simulink model "snap2_f_200msps_64i_4096c"  (R2019a)
settings: Solver=VariableStepDiscrete  StartTime=0.0  StopTime=10.0  RelTol=1e-3
undefined symbols (not defined in the file or in its folder): datetime, posixtime
libraries: xbsIndex_r4 x21354, casper_library_misc x297, casper_library_delays x19, xps_library x14, casper_library_sources x4
(part 8 of 217)

== system snap2_f_200msps_64i_4096c/version ==
  Concat : xbsIndex_r4/Concat  num_inputs=4  dbl_ovrd=off  block_type=concat
  Constant : xbsIndex_r4/Constant  const=ver_maj  gui_display_data_type=Fixed-point  arith_type=Unsigned  n_bits=8  bin_pt=0  preci_type=Single  exp_width=8  frac_width=24  explicit_period=on  period=1  equ=P=C  opselect=C  inp2=PCIN>>17  opr=+  inp1=P  carry=CIN  dbl_ovrd=off  block_type=constant
  Constant1 : xbsIndex_r4/Constant  const=ver_min  gui_display_data_type=Fixed-point  arith_type=Unsigned  n_bits=8  bin_pt=0  preci_type=Single  exp_width=8  frac_width=24  explicit_period=on  period=1  equ=P=C  opselect=C  inp2=PCIN>>17  opr=+  inp1=P  carry=CIN  dbl_ovrd=off  block_type=constant
  Constant2 : xbsIndex_r4/Constant  const=ver_rev  gui_display_data_type=Fixed-point  arith_type=Unsigned  n_bits=8  bin_pt=0  preci_type=Single  exp_width=8  frac_width=24  explicit_period=on  period=1  equ=P=C  opselect=C  inp2=PCIN>>17  opr=+  inp1=P  carry=CIN  dbl_ovrd=off  block_type=constant
  Constant3 : xbsIndex_r4/Constant  const=ver_bugfix  gui_display_data_type=Fixed-point  arith_type=Unsigned  n_bits=8  bin_pt=0  preci_type=Single  exp_width=8  frac_width=24  explicit_period=on  period=1  equ=P=C  opselect=C  inp2=PCIN>>17  opr=+  inp1=P  carry=CIN  dbl_ovrd=off  block_type=constant
  Terminator1 : Terminator
  Terminator2 : Terminator
  timestamp : Subsystem  Tag=xps:sw_reg  AncestorBlock=xps_library/Memory/software_register  mask(swreg){io_dir=To Processor, io_delay=0, init_val=0, sample_period=1, names=reg, bitwidths=32, bin_pts=0, arith_types=0, sim_port=on, show_format=off, desc_str=Unix timestamp, in integer seconds, when firmware was last compiled.}
      mask prompts: io_dir "I/O direction"; io_delay "I/O delay"; init_val "Initial Value"; sample_period "Sample period"; names "Bitfield names [msb...lsb]"; bitwidths "Bitfield widths"; bin_pts "Bitfield binary pts"; arith_types "Bitfield types, ufix=0, fix=1, bool=2"; sim_port "Provide sim input/output?"; show_format "Print format string?"; desc_str "Description"
      mask help: A 32-bit software-accessible register. Can be divided into bitfields of varying widths and types using the fields in the block mask.
      mask init:
      | swreg_init(gcb)
      settings: AttributesFormatString=1output
      mask TypeOptions io_dir: To Processor | From Processor
      mask Callback io_dir:
      | mask_enables = get_param(gcb, 'MaskEnables');
      | mask_names = get_param(gcb, 'MaskNames');
      | if strcmp(get_param(gcb, 'io_dir'), 'To Processor'),
      |     mask_enables{ismember(mask_names, 'sample_period')} = 'off';
      | else
      |     mask_enables{ismember(mask_names, 'sample_period')} = 'on';
      | end
      | set_param(gcb, 'MaskEnables', mask_enables);
      mask DialogControl ParameterTabVar0 Prompt: Setup
  unix_time : xbsIndex_r4/Constant  const=round(posixtime(datetime('now')))  gui_display_data_type=Fixed-point  arith_type=Unsigned  n_bits=32  bin_pt=0  preci_type=Single  exp_width=8  frac_width=24  explicit_period=on  period=1  equ=P=C  opselect=C  inp2=PCIN>>17  opr=+  inp1=P  carry=CIN  dbl_ovrd=off  block_type=constant
  version : Subsystem  Tag=xps:sw_reg  AncestorBlock=xps_library/Memory/software_register  mask(swreg){io_dir=To Processor, io_delay=0, init_val=0, sample_period=1, names=reg, bitwidths=32, bin_pts=0, arith_types=0, sim_port=on, show_format=off, desc_str=|}
      mask desc_str=|
      | Version register. Bits ``[31:24]``: major version. Bits
      | ``[23:16]``: minor version. Bits ``[15:8]``: revision.
      | Bits ``[7:0]``: buxfix.
      mask prompts: io_dir "I/O direction"; io_delay "I/O delay"; init_val "Initial Value"; sample_period "Sample period"; names "Bitfield names [msb...lsb]"; bitwidths "Bitfield widths"; bin_pts "Bitfield binary pts"; arith_types "Bitfield types, ufix=0, fix=1, bool=2"; sim_port "Provide sim input/output?"; show_format "Print format string?"; desc_str "Description"
      mask help: A 32-bit software-accessible register. Can be divided into bitfields of varying widths and types using the fields in the block mask.
      mask init:
      | swreg_init(gcb)
      settings: AttributesFormatString=1output
      mask TypeOptions io_dir: To Processor | From Processor
      mask Callback io_dir:
      | mask_enables = get_param(gcb, 'MaskEnables');
      | mask_names = get_param(gcb, 'MaskNames');
      | if strcmp(get_param(gcb, 'io_dir'), 'To Processor'),
      |     mask_enables{ismember(mask_names, 'sample_period')} = 'off';
      | else
      |     mask_enables{ismember(mask_names, 'sample_period')} = 'on';
      | end
      | set_param(gcb, 'MaskEnables', mask_enables);
      mask DialogControl ParameterTabVar0 Prompt: Setup
  wires:
  Constant1/1 -> Concat/2
  Concat/1 -> version/1(out_reg)
  Constant/1 -> Concat/1
  version/1(sim_out_reg) -> Terminator1/1
  Constant2/1 -> Concat/3
  Constant3/1 -> Concat/4
  timestamp/1(sim_out_reg) -> Terminator2/1
  unix_time/1 -> timestamp/1(out_reg)

== system snap2_f_200msps_64i_4096c/adc/bus_create ==
  in1 : Inport
  in2 : Inport  Port=2
  in3 : Inport  Port=3
  in4 : Inport  Port=4
  in5 : Inport  Port=5
  in6 : Inport  Port=6
  in7 : Inport  Port=7
  in8 : Inport  Port=8
  in9 : Inport  Port=9
  in10 : Inport  Port=10
  in11 : Inport  Port=11
  in12 : Inport  Port=12
  in13 : Inport  Port=13
  in14 : Inport  Port=14
  in15 : Inport  Port=15
  in16 : Inport  Port=16
  in17 : Inport  Port=17
  in18 : Inport  Port=18
  in19 : Inport  Port=19
  in20 : Inport  Port=20
  in21 : Inport  Port=21
  in22 : Inport  Port=22
  in23 : Inport  Port=23
  in24 : Inport  Port=24
  in25 : Inport  Port=25
  in26 : Inport  Port=26
  in27 : Inport  Port=27
  in28 : Inport  Port=28
  in29 : Inport  Port=29
  in30 : Inport  Port=30
  in31 : Inport  Port=31
  in32 : Inport  Port=32
  in33 : Inport  Port=33
  in34 : Inport  Port=34
  in35 : Inport  Port=35
  in36 : Inport  Port=36
  in37 : Inport  Port=37
  in38 : Inport  Port=38
  in39 : Inport  Port=39
  in40 : Inport  Port=40
  in41 : Inport  Port=41
  in42 : Inport  Port=42
  in43 : Inport  Port=43
  in44 : Inport  Port=44
  in45 : Inport  Port=45
  in46 : Inport  Port=46
  in47 : Inport  Port=47
  in48 : Inport  Port=48
  in49 : Inport  Port=49
  in50 : Inport  Port=50
  in51 : Inport  Port=51
  in52 : Inport  Port=52
  in53 : Inport  Port=53
  in54 : Inport  Port=54
  in55 : Inport  Port=55
  in56 : Inport  Port=56
  in57 : Inport  Port=57
  in58 : Inport  Port=58
  in59 : Inport  Port=59
  in60 : Inport  Port=60
  in61 : Inport  Port=61
  in62 : Inport  Port=62
  in63 : Inport  Port=63
  in64 : Inport  Port=64
  concatenate : xbsIndex_r4/Concat  num_inputs=64  dbl_ovrd=off  block_type=concat
  reinterpret{1..64} (64 alike) : xbsIndex_r4/Reinterpret  force_arith_type=on  arith_type=Unsigned  force_bin_pt=on  bin_pt=0  block_type=reinterpret
      reinterpret1 settings: infoedit="Changes signal type without altering the binary representation.   You can changed the signal between signed and unsigned, and relocate the binary point.<br><br>Hardware notes: In hardware this block costs nothing.<br><br>Example:  Suppose the input is 6 bits wide, signed, with 2 fractional bits, and the output is forced to unsigned with 0 fractional bits.  Then an input of -2.0 (1110.00 in binary 2's complement) becomes an output of 56 (111000 in binary)."
      reinterpret2 settings: infoedit="Changes signal type without altering the binary representation.   You can changed the signal between signed and unsigned, and relocate the binary point.<br><br>Hardware notes: In hardware this block costs nothing.<br><br>Example:  Suppose the input is 6 bits wide, signed, with 2 fractional bits, and the output is forced to unsigned with 0 fractional bits.  Then an input of -2.0 (1110.00 in binary 2's complement) becomes an output of 56 (111000 in binary)."
  bus_out : Outport
  wires:
  concatenate/1 -> bus_out/1
  in1/1 -> reinterpret1/1
  reinterpret1/1 -> concatenate/1
  in2/1 -> reinterpret2/1
  reinterpret2/1 -> concatenate/2
  in3/1 -> reinterpret3/1
  reinterpret3/1 -> concatenate/3
  in4/1 -> reinterpret4/1
  reinterpret4/1 -> concatenate/4
  in5/1 -> reinterpret5/1
  reinterpret5/1 -> concatenate/5
  in6/1 -> reinterpret6/1
  reinterpret6/1 -> concatenate/6
  in7/1 -> reinterpret7/1
  reinterpret7/1 -> concatenate/7
  in8/1 -> reinterpret8/1
  reinterpret8/1 -> concatenate/8
  in9/1 -> reinterpret9/1
  reinterpret9/1 -> concatenate/9
  in10/1 -> reinterpret10/1
  reinterpret10/1 -> concatenate/10
  in11/1 -> reinterpret11/1
  reinterpret11/1 -> concatenate/11
  in12/1 -> reinterpret12/1
  reinterpret12/1 -> concatenate/12
  in13/1 -> reinterpret13/1
  reinterpret13/1 -> concatenate/13
  in14/1 -> reinterpret14/1
  reinterpret14/1 -> concatenate/14
  in15/1 -> reinterpret15/1
  reinterpret15/1 -> concatenate/15
  in16/1 -> reinterpret16/1
  reinterpret16/1 -> concatenate/16
  in17/1 -> reinterpret17/1
  reinterpret17/1 -> concatenate/17
  in18/1 -> reinterpret18/1
  reinterpret18/1 -> concatenate/18
  in19/1 -> reinterpret19/1
  reinterpret19/1 -> concatenate/19
  in20/1 -> reinterpret20/1
  reinterpret20/1 -> concatenate/20
  in21/1 -> reinterpret21/1
  reinterpret21/1 -> concatenate/21
  in22/1 -> reinterpret22/1
  reinterpret22/1 -> concatenate/22
  in23/1 -> reinterpret23/1
  reinterpret23/1 -> concatenate/23
  in24/1 -> reinterpret24/1
  reinterpret24/1 -> concatenate/24
  in25/1 -> reinterpret25/1
  reinterpret25/1 -> concatenate/25
  in26/1 -> reinterpret26/1
  reinterpret26/1 -> concatenate/26
  in27/1 -> reinterpret27/1
  reinterpret27/1 -> concatenate/27
  in28/1 -> reinterpret28/1
  reinterpret28/1 -> concatenate/28
  in29/1 -> reinterpret29/1
  reinterpret29/1 -> concatenate/29
  in30/1 -> reinterpret30/1
  reinterpret30/1 -> concatenate/30
  in31/1 -> reinterpret31/1
  reinterpret31/1 -> concatenate/31
  in32/1 -> reinterpret32/1
  reinterpret32/1 -> concatenate/32
  in33/1 -> reinterpret33/1
  reinterpret33/1 -> concatenate/33
  in34/1 -> reinterpret34/1
  reinterpret34/1 -> concatenate/34
  in35/1 -> reinterpret35/1
  reinterpret35/1 -> concatenate/35
  in36/1 -> reinterpret36/1
  reinterpret36/1 -> concatenate/36
  in37/1 -> reinterpret37/1
  reinterpret37/1 -> concatenate/37
  in38/1 -> reinterpret38/1
  reinterpret38/1 -> concatenate/38
  in39/1 -> reinterpret39/1
  reinterpret39/1 -> concatenate/39
  in40/1 -> reinterpret40/1
  reinterpret40/1 -> concatenate/40
  in41/1 -> reinterpret41/1
  reinterpret41/1 -> concatenate/41
  in42/1 -> reinterpret42/1
  reinterpret42/1 -> concatenate/42
  in43/1 -> reinterpret43/1
  reinterpret43/1 -> concatenate/43
  in44/1 -> reinterpret44/1
  reinterpret44/1 -> concatenate/44
  in45/1 -> reinterpret45/1
  reinterpret45/1 -> concatenate/45
  in46/1 -> reinterpret46/1
  reinterpret46/1 -> concatenate/46
  in47/1 -> reinterpret47/1
  reinterpret47/1 -> concatenate/47
  in48/1 -> reinterpret48/1
  reinterpret48/1 -> concatenate/48
  in49/1 -> reinterpret49/1
  reinterpret49/1 -> concatenate/49
  in50/1 -> reinterpret50/1
  reinterpret50/1 -> concatenate/50
  in51/1 -> reinterpret51/1
  reinterpret51/1 -> concatenate/51
  in52/1 -> reinterpret52/1
  reinterpret52/1 -> concatenate/52
  in53/1 -> reinterpret53/1
  reinterpret53/1 -> concatenate/53
  in54/1 -> reinterpret54/1
  reinterpret54/1 -> concatenate/54
  in55/1 -> reinterpret55/1
  reinterpret55/1 -> concatenate/55
  in56/1 -> reinterpret56/1
  reinterpret56/1 -> concatenate/56
  in57/1 -> reinterpret57/1
  reinterpret57/1 -> concatenate/57
  in58/1 -> reinterpret58/1
  reinterpret58/1 -> concatenate/58
  in59/1 -> reinterpret59/1
  reinterpret59/1 -> concatenate/59
  in60/1 -> reinterpret60/1
  reinterpret60/1 -> concatenate/60
  in61/1 -> reinterpret61/1
  reinterpret61/1 -> concatenate/61
  in62/1 -> reinterpret62/1
  reinterpret62/1 -> concatenate/62
  in63/1 -> reinterpret63/1
  reinterpret63/1 -> concatenate/63
  in64/1 -> reinterpret64/1
  reinterpret64/1 -> concatenate/64

== system snap2_f_200msps_64i_4096c/adc/fmc0 ==
  a1_sim : Inport
  a2_sim : Inport  Port=2
  a3_sim : Inport  Port=3
  a4_sim : Inport  Port=4
  b1_sim : Inport  Port=5
  b2_sim : Inport  Port=6
  b3_sim : Inport  Port=7
  b4_sim : Inport  Port=8
  c1_sim : Inport  Port=9
  c2_sim : Inport  Port=10
  c3_sim : Inport  Port=11
  c4_sim : Inport  Port=12
  d1_sim : Inport  Port=13
  d2_sim : Inport  Port=14
  d3_sim : Inport  Port=15
  d4_sim : Inport  Port=16
  e1_sim : Inport  Port=17
  e2_sim : Inport  Port=18
  e3_sim : Inport  Port=19
  e4_sim : Inport  Port=20
  f1_sim : Inport  Port=21
  f2_sim : Inport  Port=22
  f3_sim : Inport  Port=23
  f4_sim : Inport  Port=24
  g1_sim : Inport  Port=25
  g2_sim : Inport  Port=26
  g3_sim : Inport  Port=27
  g4_sim : Inport  Port=28
  h1_sim : Inport  Port=29
  h2_sim : Inport  Port=30
  h3_sim : Inport  Port=31
  h4_sim : Inport  Port=32
  sync : Inport  Port=33
  snapshot_trig : Inport  Port=34
  sim_sync_out : Inport  Port=35
  rst : Inport  Port=36
  rst_term : Terminator
  snap2_f_200msps_64i_4096c_adc_fmc0_a{1..4} (4 alike) : xbsIndex_r4/Gateway In  gui_display_data_type=Fixed-point  arith_type="Signed  (2's comp)"  n_bits=10  bin_pt=9  preci_type=Single  exp_width=8  frac_width=24  rows=1  columns=1  quantization="Round  (unbiased: +/- Inf)"  overflow=Saturate  period=1  UseAsADC=off  ADCChannel='1'  interface=None  automatic_assignment=on  address_offset=hex2dec('00')  intf_name=''  intf_description=''  default_value=0  timing_constraint=None  locs_specified=off  LOCs={}  io_standard={}  inherit_from_input=off  hdl_port=on  dbl_ovrd=off  block_type=gatewayin
  snap2_f_200msps_64i_4096c_adc_fmc0_adc_rst : xbsIndex_r4/Gateway Out  inherit_from_input=off  hdl_port=on  rows=1  columns=1  UseAsDAC=off  DACChannel='1'  interface=None  automatic_assignment=on  address_offset=hex2dec('00')  intf_name=''  intf_description=''  timing_constraint=None  locs_specified=off  LOCs={}  io_standard={}  block_type=gatewayout
  snap2_f_200msps_64i_4096c_adc_fmc0_adc_sync : xbsIndex_r4/Gateway Out  inherit_from_input=off  hdl_port=on  rows=1  columns=1  UseAsDAC=off  DACChannel='1'  interface=None  automatic_assignment=on  address_offset=hex2dec('00')  intf_name=''  intf_description=''  timing_constraint=None  locs_specified=off  LOCs={}  io_standard={}  block_type=gatewayout
  snap2_f_200msps_64i_4096c_adc_fmc0_adc_sync_out : xbsIndex_r4/Gateway In  gui_display_data_type=Fixed-point  arith_type=Boolean  n_bits=16  bin_pt=14  preci_type=Single  exp_width=8  frac_width=24  rows=1  columns=1  quantization="Round  (unbiased: +/- Inf)"  overflow=Saturate  period=1  UseAsADC=off  ADCChannel='1'  interface=None  automatic_assignment=on  address_offset=hex2dec('00')  intf_name=''  intf_description=''  default_value=0  timing_constraint=None  locs_specified=off  LOCs={}  io_standard={}  inherit_from_input=off  hdl_port=on  dbl_ovrd=off  block_type=gatewayin
  snap2_f_200msps_64i_4096c_adc_fmc0_b{1..4} (4 alike) : xbsIndex_r4/Gateway In  gui_display_data_type=Fixed-point  arith_type="Signed  (2's comp)"  n_bits=10  bin_pt=9  preci_type=Single  exp_width=8  frac_width=24  rows=1  columns=1  quantization="Round  (unbiased: +/- Inf)"  overflow=Saturate  period=1  UseAsADC=off  ADCChannel='1'  interface=None  automatic_assignment=on  address_offset=hex2dec('00')  intf_name=''  intf_description=''  default_value=0  timing_constraint=None  locs_specified=off  LOCs={}  io_standard={}  inherit_from_input=off  hdl_port=on  dbl_ovrd=off  block_type=gatewayin
  snap2_f_200msps_64i_4096c_adc_fmc0_c{1..4} (4 alike) : xbsIndex_r4/Gateway In  gui_display_data_type=Fixed-point  arith_type="Signed  (2's comp)"  n_bits=10  bin_pt=9  preci_type=Single  exp_width=8  frac_width=24  rows=1  columns=1  quantization="Round  (unbiased: +/- Inf)"  overflow=Saturate  period=1  UseAsADC=off  ADCChannel='1'  interface=None  automatic_assignment=on  address_offset=hex2dec('00')  intf_name=''  intf_description=''  default_value=0  timing_constraint=None  locs_specified=off  LOCs={}  io_standard={}  inherit_from_input=off  hdl_port=on  dbl_ovrd=off  block_type=gatewayin
  snap2_f_200msps_64i_4096c_adc_fmc0_d{1..4} (4 alike) : xbsIndex_r4/Gateway In  gui_display_data_type=Fixed-point  arith_type="Signed  (2's comp)"  n_bits=10  bin_pt=9  preci_type=Single  exp_width=8  frac_width=24  rows=1  columns=1  quantization="Round  (unbiased: +/- Inf)"  overflow=Saturate  period=1  UseAsADC=off  ADCChannel='1'  interface=None  automatic_assignment=on  address_offset=hex2dec('00')  intf_name=''  intf_description=''  default_value=0  timing_constraint=None  locs_specified=off  LOCs={}  io_standard={}  inherit_from_input=off  hdl_port=on  dbl_ovrd=off  block_type=gatewayin
  snap2_f_200msps_64i_4096c_adc_fmc0_e{1..4} (4 alike) : xbsIndex_r4/Gateway In  gui_display_data_type=Fixed-point  arith_type="Signed  (2's comp)"  n_bits=10  bin_pt=9  preci_type=Single  exp_width=8  frac_width=24  rows=1  columns=1  quantization="Round  (unbiased: +/- Inf)"  overflow=Saturate  period=1  UseAsADC=off  ADCChannel='1'  interface=None  automatic_assignment=on  address_offset=hex2dec('00')  intf_name=''  intf_description=''  default_value=0  timing_constraint=None  locs_specified=off  LOCs={}  io_standard={}  inherit_from_input=off  hdl_port=on  dbl_ovrd=off  block_type=gatewayin
  snap2_f_200msps_64i_4096c_adc_fmc0_f{1..4} (4 alike) : xbsIndex_r4/Gateway In  gui_display_data_type=Fixed-point  arith_type="Signed  (2's comp)"  n_bits=10  bin_pt=9  preci_type=Single  exp_width=8  frac_width=24  rows=1  columns=1  quantization="Round  (unbiased: +/- Inf)"  overflow=Saturate  period=1  UseAsADC=off  ADCChannel='1'  interface=None  automatic_assignment=on  address_offset=hex2dec('00')  intf_name=''  intf_description=''  default_value=0  timing_constraint=None  locs_specified=off  LOCs={}  io_standard={}  inherit_from_input=off  hdl_port=on  dbl_ovrd=off  block_type=gatewayin
  snap2_f_200msps_64i_4096c_adc_fmc0_g{1..4} (4 alike) : xbsIndex_r4/Gateway In  gui_display_data_type=Fixed-point  arith_type="Signed  (2's comp)"  n_bits=10  bin_pt=9  preci_type=Single  exp_width=8  frac_width=24  rows=1  columns=1  quantization="Round  (unbiased: +/- Inf)"  overflow=Saturate  period=1  UseAsADC=off  ADCChannel='1'  interface=None  automatic_assignment=on  address_offset=hex2dec('00')  intf_name=''  intf_description=''  default_value=0  timing_constraint=None  locs_specified=off  LOCs={}  io_standard={}  inherit_from_input=off  hdl_port=on  dbl_ovrd=off  block_type=gatewayin
  snap2_f_200msps_64i_4096c_adc_fmc0_h{1..4} (4 alike) : xbsIndex_r4/Gateway In  gui_display_data_type=Fixed-point  arith_type="Signed  (2's comp)"  n_bits=10  bin_pt=9  preci_type=Single  exp_width=8  frac_width=24  rows=1  columns=1  quantization="Round  (unbiased: +/- Inf)"  overflow=Saturate  period=1  UseAsADC=off  ADCChannel='1'  interface=None  automatic_assignment=on  address_offset=hex2dec('00')  intf_name=''  intf_description=''  default_value=0  timing_constraint=None  locs_specified=off  LOCs={}  io_standard={}  inherit_from_input=off  hdl_port=on  dbl_ovrd=off  block_type=gatewayin
  snap2_f_200msps_64i_4096c_adc_fmc0_snapshot_ext_trigger : xbsIndex_r4/Gateway Out  inherit_from_input=off  hdl_port=on  rows=1  columns=1  UseAsDAC=off  DACChannel='1'  interface=None  automatic_assignment=on  address_offset=hex2dec('00')  intf_name=''  intf_description=''  timing_constraint=None  locs_specified=off  LOCs={}  io_standard={}  block_type=gatewayout
  snapshot_trig_term : Terminator
  sync_term : Terminator
  a1 : Outport
  a2 : Outport  Port=2
  a3 : Outport  Port=3
  a4 : Outport  Port=4
  b1 : Outport  Port=5
  b2 : Outport  Port=6
  b3 : Outport  Port=7
  b4 : Outport  Port=8
  c1 : Outport  Port=9
  c2 : Outport  Port=10
  c3 : Outport  Port=11
  c4 : Outport  Port=12
  d1 : Outport  Port=13
  d2 : Outport  Port=14
  d3 : Outport  Port=15
  d4 : Outport  Port=16
  e1 : Outport  Port=17
  e2 : Outport  Port=18
  e3 : Outport  Port=19
  e4 : Outport  Port=20
  f1 : Outport  Port=21
  f2 : Outport  Port=22
  f3 : Outport  Port=23
  f4 : Outport  Port=24
  g1 : Outport  Port=25
  g2 : Outport  Port=26
  g3 : Outport  Port=27
  g4 : Outport  Port=28
  h1 : Outport  Port=29
  h2 : Outport  Port=30
  h3 : Outport  Port=31
  h4 : Outport  Port=32
  sync_out : Outport  Port=33
  wires:
  a1_sim/1 -> snap2_f_200msps_64i_4096c_adc_fmc0_a1/1
  snap2_f_200msps_64i_4096c_adc_fmc0_a1/1 -> a1/1  "a1"
  a2_sim/1 -> snap2_f_200msps_64i_4096c_adc_fmc0_a2/1
  snap2_f_200msps_64i_4096c_adc_fmc0_a2/1 -> a2/1  "a2"
  a3_sim/1 -> snap2_f_200msps_64i_4096c_adc_fmc0_a3/1
  snap2_f_200msps_64i_4096c_adc_fmc0_a3/1 -> a3/1  "a3"
  a4_sim/1 -> snap2_f_200msps_64i_4096c_adc_fmc0_a4/1
  snap2_f_200msps_64i_4096c_adc_fmc0_a4/1 -> a4/1  "a4"
  b1_sim/1 -> snap2_f_200msps_64i_4096c_adc_fmc0_b1/1
  snap2_f_200msps_64i_4096c_adc_fmc0_b1/1 -> b1/1  "b1"
  b2_sim/1 -> snap2_f_200msps_64i_4096c_adc_fmc0_b2/1
  snap2_f_200msps_64i_4096c_adc_fmc0_b2/1 -> b2/1  "b2"
  b3_sim/1 -> snap2_f_200msps_64i_4096c_adc_fmc0_b3/1
  snap2_f_200msps_64i_4096c_adc_fmc0_b3/1 -> b3/1  "b3"
  b4_sim/1 -> snap2_f_200msps_64i_4096c_adc_fmc0_b4/1
  snap2_f_200msps_64i_4096c_adc_fmc0_b4/1 -> b4/1  "b4"
  c1_sim/1 -> snap2_f_200msps_64i_4096c_adc_fmc0_c1/1
  snap2_f_200msps_64i_4096c_adc_fmc0_c1/1 -> c1/1  "c1"
  c2_sim/1 -> snap2_f_200msps_64i_4096c_adc_fmc0_c2/1
  snap2_f_200msps_64i_4096c_adc_fmc0_c2/1 -> c2/1  "c2"
  c3_sim/1 -> snap2_f_200msps_64i_4096c_adc_fmc0_c3/1
  snap2_f_200msps_64i_4096c_adc_fmc0_c3/1 -> c3/1  "c3"
  c4_sim/1 -> snap2_f_200msps_64i_4096c_adc_fmc0_c4/1
  snap2_f_200msps_64i_4096c_adc_fmc0_c4/1 -> c4/1  "c4"
  d1_sim/1 -> snap2_f_200msps_64i_4096c_adc_fmc0_d1/1
  snap2_f_200msps_64i_4096c_adc_fmc0_d1/1 -> d1/1  "d1"
  d2_sim/1 -> snap2_f_200msps_64i_4096c_adc_fmc0_d2/1
  snap2_f_200msps_64i_4096c_adc_fmc0_d2/1 -> d2/1  "d2"
  d3_sim/1 -> snap2_f_200msps_64i_4096c_adc_fmc0_d3/1
  snap2_f_200msps_64i_4096c_adc_fmc0_d3/1 -> d3/1  "d3"
  d4_sim/1 -> snap2_f_200msps_64i_4096c_adc_fmc0_d4/1
  snap2_f_200msps_64i_4096c_adc_fmc0_d4/1 -> d4/1  "d4"
  e1_sim/1 -> snap2_f_200msps_64i_4096c_adc_fmc0_e1/1
  snap2_f_200msps_64i_4096c_adc_fmc0_e1/1 -> e1/1  "e1"
  e2_sim/1 -> snap2_f_200msps_64i_4096c_adc_fmc0_e2/1
  snap2_f_200msps_64i_4096c_adc_fmc0_e2/1 -> e2/1  "e2"
  e3_sim/1 -> snap2_f_200msps_64i_4096c_adc_fmc0_e3/1
  snap2_f_200msps_64i_4096c_adc_fmc0_e3/1 -> e3/1  "e3"
  e4_sim/1 -> snap2_f_200msps_64i_4096c_adc_fmc0_e4/1
  snap2_f_200msps_64i_4096c_adc_fmc0_e4/1 -> e4/1  "e4"
  f1_sim/1 -> snap2_f_200msps_64i_4096c_adc_fmc0_f1/1
  snap2_f_200msps_64i_4096c_adc_fmc0_f1/1 -> f1/1  "f1"
  f2_sim/1 -> snap2_f_200msps_64i_4096c_adc_fmc0_f2/1
  snap2_f_200msps_64i_4096c_adc_fmc0_f2/1 -> f2/1  "f2"
  f3_sim/1 -> snap2_f_200msps_64i_4096c_adc_fmc0_f3/1
  snap2_f_200msps_64i_4096c_adc_fmc0_f3/1 -> f3/1  "f3"
  f4_sim/1 -> snap2_f_200msps_64i_4096c_adc_fmc0_f4/1
  snap2_f_200msps_64i_4096c_adc_fmc0_f4/1 -> f4/1  "f4"
  g1_sim/1 -> snap2_f_200msps_64i_4096c_adc_fmc0_g1/1
  snap2_f_200msps_64i_4096c_adc_fmc0_g1/1 -> g1/1  "g1"
  g2_sim/1 -> snap2_f_200msps_64i_4096c_adc_fmc0_g2/1
  snap2_f_200msps_64i_4096c_adc_fmc0_g2/1 -> g2/1  "g2"
  g3_sim/1 -> snap2_f_200msps_64i_4096c_adc_fmc0_g3/1
  snap2_f_200msps_64i_4096c_adc_fmc0_g3/1 -> g3/1  "g3"
  g4_sim/1 -> snap2_f_200msps_64i_4096c_adc_fmc0_g4/1
  snap2_f_200msps_64i_4096c_adc_fmc0_g4/1 -> g4/1  "g4"
  h1_sim/1 -> snap2_f_200msps_64i_4096c_adc_fmc0_h1/1
  snap2_f_200msps_64i_4096c_adc_fmc0_h1/1 -> h1/1  "h1"
  h2_sim/1 -> snap2_f_200msps_64i_4096c_adc_fmc0_h2/1
  snap2_f_200msps_64i_4096c_adc_fmc0_h2/1 -> h2/1  "h2"
  h3_sim/1 -> snap2_f_200msps_64i_4096c_adc_fmc0_h3/1
  snap2_f_200msps_64i_4096c_adc_fmc0_h3/1 -> h3/1  "h3"
  h4_sim/1 -> snap2_f_200msps_64i_4096c_adc_fmc0_h4/1
  snap2_f_200msps_64i_4096c_adc_fmc0_h4/1 -> h4/1  "h4"
  sync/1 -> snap2_f_200msps_64i_4096c_adc_fmc0_adc_sync/1
  snap2_f_200msps_64i_4096c_adc_fmc0_adc_sync/1 -> sync_term/1
  rst/1 -> snap2_f_200msps_64i_4096c_adc_fmc0_adc_rst/1
  snap2_f_200msps_64i_4096c_adc_fmc0_adc_rst/1 -> rst_term/1
  snapshot_trig/1 -> snap2_f_200msps_64i_4096c_adc_fmc0_snapshot_ext_trigger/1
  snap2_f_200msps_64i_4096c_adc_fmc0_snapshot_ext_trigger/1 -> snapshot_trig_term/1
  sim_sync_out/1 -> snap2_f_200msps_64i_4096c_adc_fmc0_adc_sync_out/1
  snap2_f_200msps_64i_4096c_adc_fmc0_adc_sync_out/1 -> sync_out/1

== system snap2_f_200msps_64i_4096c/adc/fmc1 ==
  a1_sim : Inport
  a2_sim : Inport  Port=2
  a3_sim : Inport  Port=3
  a4_sim : Inport  Port=4
  b1_sim : Inport  Port=5
  b2_sim : Inport  Port=6
  b3_sim : Inport  Port=7
  b4_sim : Inport  Port=8
  c1_sim : Inport  Port=9
  c2_sim : Inport  Port=10
  c3_sim : Inport  Port=11
  c4_sim : Inport  Port=12
  d1_sim : Inport  Port=13
  d2_sim : Inport  Port=14
  d3_sim : Inport  Port=15
  d4_sim : Inport  Port=16
  e1_sim : Inport  Port=17
  e2_sim : Inport  Port=18
  e3_sim : Inport  Port=19
  e4_sim : Inport  Port=20
  f1_sim : Inport  Port=21
  f2_sim : Inport  Port=22
  f3_sim : Inport  Port=23
  f4_sim : Inport  Port=24
  g1_sim : Inport  Port=25
  g2_sim : Inport  Port=26
  g3_sim : Inport  Port=27
  g4_sim : Inport  Port=28
  h1_sim : Inport  Port=29
  h2_sim : Inport  Port=30
  h3_sim : Inport  Port=31
  h4_sim : Inport  Port=32
  sync : Inport  Port=33
  snapshot_trig : Inport  Port=34
  sim_sync_out : Inport  Port=35
  rst : Inport  Port=36
  rst_term : Terminator
  snap2_f_200msps_64i_4096c_adc_fmc1_a{1..4} (4 alike) : xbsIndex_r4/Gateway In  gui_display_data_type=Fixed-point  arith_type="Signed  (2's comp)"  n_bits=10  bin_pt=9  preci_type=Single  exp_width=8  frac_width=24  rows=1  columns=1  quantization="Round  (unbiased: +/- Inf)"  overflow=Saturate  period=1  UseAsADC=off  ADCChannel='1'  interface=None  automatic_assignment=on  address_offset=hex2dec('00')  intf_name=''  intf_description=''  default_value=0  timing_constraint=None  locs_specified=off  LOCs={}  io_standard={}  inherit_from_input=off  hdl_port=on  dbl_ovrd=off  block_type=gatewayin
  snap2_f_200msps_64i_4096c_adc_fmc1_adc_rst : xbsIndex_r4/Gateway Out  inherit_from_input=off  hdl_port=on  rows=1  columns=1  UseAsDAC=off  DACChannel='1'  interface=None  automatic_assignment=on  address_offset=hex2dec('00')  intf_name=''  intf_description=''  timing_constraint=None  locs_specified=off  LOCs={}  io_standard={}  block_type=gatewayout
  snap2_f_200msps_64i_4096c_adc_fmc1_adc_sync : xbsIndex_r4/Gateway Out  inherit_from_input=off  hdl_port=on  rows=1  columns=1  UseAsDAC=off  DACChannel='1'  interface=None  automatic_assignment=on  address_offset=hex2dec('00')  intf_name=''  intf_description=''  timing_constraint=None  locs_specified=off  LOCs={}  io_standard={}  block_type=gatewayout
  snap2_f_200msps_64i_4096c_adc_fmc1_adc_sync_out : xbsIndex_r4/Gateway In  gui_display_data_type=Fixed-point  arith_type=Boolean  n_bits=16  bin_pt=14  preci_type=Single  exp_width=8  frac_width=24  rows=1  columns=1  quantization="Round  (unbiased: +/- Inf)"  overflow=Saturate  period=1  UseAsADC=off  ADCChannel='1'  interface=None  automatic_assignment=on  address_offset=hex2dec('00')  intf_name=''  intf_description=''  default_value=0  timing_constraint=None  locs_specified=off  LOCs={}  io_standard={}  inherit_from_input=off  hdl_port=on  dbl_ovrd=off  block_type=gatewayin
  snap2_f_200msps_64i_4096c_adc_fmc1_b{1..4} (4 alike) : xbsIndex_r4/Gateway In  gui_display_data_type=Fixed-point  arith_type="Signed  (2's comp)"  n_bits=10  bin_pt=9  preci_type=Single  exp_width=8  frac_width=24  rows=1  columns=1  quantization="Round  (unbiased: +/- Inf)"  overflow=Saturate  period=1  UseAsADC=off  ADCChannel='1'  interface=None  automatic_assignment=on  address_offset=hex2dec('00')  intf_name=''  intf_description=''  default_value=0  timing_constraint=None  locs_specified=off  LOCs={}  io_standard={}  inherit_from_input=off  hdl_port=on  dbl_ovrd=off  block_type=gatewayin
  snap2_f_200msps_64i_4096c_adc_fmc1_c{1..4} (4 alike) : xbsIndex_r4/Gateway In  gui_display_data_type=Fixed-point  arith_type="Signed  (2's comp)"  n_bits=10  bin_pt=9  preci_type=Single  exp_width=8  frac_width=24  rows=1  columns=1  quantization="Round  (unbiased: +/- Inf)"  overflow=Saturate  period=1  UseAsADC=off  ADCChannel='1'  interface=None  automatic_assignment=on  address_offset=hex2dec('00')  intf_name=''  intf_description=''  default_value=0  timing_constraint=None  locs_specified=off  LOCs={}  io_standard={}  inherit_from_input=off  hdl_port=on  dbl_ovrd=off  block_type=gatewayin
  snap2_f_200msps_64i_4096c_adc_fmc1_d{1..4} (4 alike) : xbsIndex_r4/Gateway In  gui_display_data_type=Fixed-point  arith_type="Signed  (2's comp)"  n_bits=10  bin_pt=9  preci_type=Single  exp_width=8  frac_width=24  rows=1  columns=1  quantization="Round  (unbiased: +/- Inf)"  overflow=Saturate  period=1  UseAsADC=off  ADCChannel='1'  interface=None  automatic_assignment=on  address_offset=hex2dec('00')  intf_name=''  intf_description=''  default_value=0  timing_constraint=None  locs_specified=off  LOCs={}  io_standard={}  inherit_from_input=off  hdl_port=on  dbl_ovrd=off  block_type=gatewayin
  snap2_f_200msps_64i_4096c_adc_fmc1_e{1..4} (4 alike) : xbsIndex_r4/Gateway In  gui_display_data_type=Fixed-point  arith_type="Signed  (2's comp)"  n_bits=10  bin_pt=9  preci_type=Single  exp_width=8  frac_width=24  rows=1  columns=1  quantization="Round  (unbiased: +/- Inf)"  overflow=Saturate  period=1  UseAsADC=off  ADCChannel='1'  interface=None  automatic_assignment=on  address_offset=hex2dec('00')  intf_name=''  intf_description=''  default_value=0  timing_constraint=None  locs_specified=off  LOCs={}  io_standard={}  inherit_from_input=off  hdl_port=on  dbl_ovrd=off  block_type=gatewayin
  snap2_f_200msps_64i_4096c_adc_fmc1_f{1..4} (4 alike) : xbsIndex_r4/Gateway In  gui_display_data_type=Fixed-point  arith_type="Signed  (2's comp)"  n_bits=10  bin_pt=9  preci_type=Single  exp_width=8  frac_width=24  rows=1  columns=1  quantization="Round  (unbiased: +/- Inf)"  overflow=Saturate  period=1  UseAsADC=off  ADCChannel='1'  interface=None  automatic_assignment=on  address_offset=hex2dec('00')  intf_name=''  intf_description=''  default_value=0  timing_constraint=None  locs_specified=off  LOCs={}  io_standard={}  inherit_from_input=off  hdl_port=on  dbl_ovrd=off  block_type=gatewayin
  snap2_f_200msps_64i_4096c_adc_fmc1_g{1..4} (4 alike) : xbsIndex_r4/Gateway In  gui_display_data_type=Fixed-point  arith_type="Signed  (2's comp)"  n_bits=10  bin_pt=9  preci_type=Single  exp_width=8  frac_width=24  rows=1  columns=1  quantization="Round  (unbiased: +/- Inf)"  overflow=Saturate  period=1  UseAsADC=off  ADCChannel='1'  interface=None  automatic_assignment=on  address_offset=hex2dec('00')  intf_name=''  intf_description=''  default_value=0  timing_constraint=None  locs_specified=off  LOCs={}  io_standard={}  inherit_from_input=off  hdl_port=on  dbl_ovrd=off  block_type=gatewayin
  snap2_f_200msps_64i_4096c_adc_fmc1_h{1..4} (4 alike) : xbsIndex_r4/Gateway In  gui_display_data_type=Fixed-point  arith_type="Signed  (2's comp)"  n_bits=10  bin_pt=9  preci_type=Single  exp_width=8  frac_width=24  rows=1  columns=1  quantization="Round  (unbiased: +/- Inf)"  overflow=Saturate  period=1  UseAsADC=off  ADCChannel='1'  interface=None  automatic_assignment=on  address_offset=hex2dec('00')  intf_name=''  intf_description=''  default_value=0  timing_constraint=None  locs_specified=off  LOCs={}  io_standard={}  inherit_from_input=off  hdl_port=on  dbl_ovrd=off  block_type=gatewayin
  snap2_f_200msps_64i_4096c_adc_fmc1_snapshot_ext_trigger : xbsIndex_r4/Gateway Out  inherit_from_input=off  hdl_port=on  rows=1  columns=1  UseAsDAC=off  DACChannel='1'  interface=None  automatic_assignment=on  address_offset=hex2dec('00')  intf_name=''  intf_description=''  timing_constraint=None  locs_specified=off  LOCs={}  io_standard={}  block_type=gatewayout
  snapshot_trig_term : Terminator
  sync_term : Terminator
  a1 : Outport
  a2 : Outport  Port=2
  a3 : Outport  Port=3
  a4 : Outport  Port=4
  b1 : Outport  Port=5
  b2 : Outport  Port=6
  b3 : Outport  Port=7
  b4 : Outport  Port=8
  c1 : Outport  Port=9
  c2 : Outport  Port=10
  c3 : Outport  Port=11
  c4 : Outport  Port=12
  d1 : Outport  Port=13
  d2 : Outport  Port=14
  d3 : Outport  Port=15
  d4 : Outport  Port=16
  e1 : Outport  Port=17
  e2 : Outport  Port=18
  e3 : Outport  Port=19
  e4 : Outport  Port=20
  f1 : Outport  Port=21
  f2 : Outport  Port=22
  f3 : Outport  Port=23
  f4 : Outport  Port=24
  g1 : Outport  Port=25
  g2 : Outport  Port=26
  g3 : Outport  Port=27
  g4 : Outport  Port=28
  h1 : Outport  Port=29
  h2 : Outport  Port=30
  h3 : Outport  Port=31
  h4 : Outport  Port=32
  sync_out : Outport  Port=33
  wires:
  a1_sim/1 -> snap2_f_200msps_64i_4096c_adc_fmc1_a1/1
  snap2_f_200msps_64i_4096c_adc_fmc1_a1/1 -> a1/1  "a1"
  a2_sim/1 -> snap2_f_200msps_64i_4096c_adc_fmc1_a2/1
  snap2_f_200msps_64i_4096c_adc_fmc1_a2/1 -> a2/1  "a2"
  a3_sim/1 -> snap2_f_200msps_64i_4096c_adc_fmc1_a3/1
  snap2_f_200msps_64i_4096c_adc_fmc1_a3/1 -> a3/1  "a3"
  a4_sim/1 -> snap2_f_200msps_64i_4096c_adc_fmc1_a4/1
  snap2_f_200msps_64i_4096c_adc_fmc1_a4/1 -> a4/1  "a4"
  b1_sim/1 -> snap2_f_200msps_64i_4096c_adc_fmc1_b1/1
  snap2_f_200msps_64i_4096c_adc_fmc1_b1/1 -> b1/1  "b1"
  b2_sim/1 -> snap2_f_200msps_64i_4096c_adc_fmc1_b2/1
  snap2_f_200msps_64i_4096c_adc_fmc1_b2/1 -> b2/1  "b2"
  b3_sim/1 -> snap2_f_200msps_64i_4096c_adc_fmc1_b3/1
  snap2_f_200msps_64i_4096c_adc_fmc1_b3/1 -> b3/1  "b3"
  b4_sim/1 -> snap2_f_200msps_64i_4096c_adc_fmc1_b4/1
  snap2_f_200msps_64i_4096c_adc_fmc1_b4/1 -> b4/1  "b4"
  c1_sim/1 -> snap2_f_200msps_64i_4096c_adc_fmc1_c1/1
  snap2_f_200msps_64i_4096c_adc_fmc1_c1/1 -> c1/1  "c1"
  c2_sim/1 -> snap2_f_200msps_64i_4096c_adc_fmc1_c2/1
  snap2_f_200msps_64i_4096c_adc_fmc1_c2/1 -> c2/1  "c2"
  c3_sim/1 -> snap2_f_200msps_64i_4096c_adc_fmc1_c3/1
  snap2_f_200msps_64i_4096c_adc_fmc1_c3/1 -> c3/1  "c3"
  c4_sim/1 -> snap2_f_200msps_64i_4096c_adc_fmc1_c4/1
  snap2_f_200msps_64i_4096c_adc_fmc1_c4/1 -> c4/1  "c4"
  d1_sim/1 -> snap2_f_200msps_64i_4096c_adc_fmc1_d1/1
  snap2_f_200msps_64i_4096c_adc_fmc1_d1/1 -> d1/1  "d1"
  d2_sim/1 -> snap2_f_200msps_64i_4096c_adc_fmc1_d2/1
  snap2_f_200msps_64i_4096c_adc_fmc1_d2/1 -> d2/1  "d2"
  d3_sim/1 -> snap2_f_200msps_64i_4096c_adc_fmc1_d3/1
  snap2_f_200msps_64i_4096c_adc_fmc1_d3/1 -> d3/1  "d3"
  d4_sim/1 -> snap2_f_200msps_64i_4096c_adc_fmc1_d4/1
  snap2_f_200msps_64i_4096c_adc_fmc1_d4/1 -> d4/1  "d4"
  e1_sim/1 -> snap2_f_200msps_64i_4096c_adc_fmc1_e1/1
  snap2_f_200msps_64i_4096c_adc_fmc1_e1/1 -> e1/1  "e1"
  e2_sim/1 -> snap2_f_200msps_64i_4096c_adc_fmc1_e2/1
  snap2_f_200msps_64i_4096c_adc_fmc1_e2/1 -> e2/1  "e2"
  e3_sim/1 -> snap2_f_200msps_64i_4096c_adc_fmc1_e3/1
  snap2_f_200msps_64i_4096c_adc_fmc1_e3/1 -> e3/1  "e3"
  e4_sim/1 -> snap2_f_200msps_64i_4096c_adc_fmc1_e4/1
  snap2_f_200msps_64i_4096c_adc_fmc1_e4/1 -> e4/1  "e4"
  f1_sim/1 -> snap2_f_200msps_64i_4096c_adc_fmc1_f1/1
  snap2_f_200msps_64i_4096c_adc_fmc1_f1/1 -> f1/1  "f1"
  f2_sim/1 -> snap2_f_200msps_64i_4096c_adc_fmc1_f2/1
  snap2_f_200msps_64i_4096c_adc_fmc1_f2/1 -> f2/1  "f2"
  f3_sim/1 -> snap2_f_200msps_64i_4096c_adc_fmc1_f3/1
  snap2_f_200msps_64i_4096c_adc_fmc1_f3/1 -> f3/1  "f3"
  f4_sim/1 -> snap2_f_200msps_64i_4096c_adc_fmc1_f4/1
  snap2_f_200msps_64i_4096c_adc_fmc1_f4/1 -> f4/1  "f4"
  g1_sim/1 -> snap2_f_200msps_64i_4096c_adc_fmc1_g1/1
  snap2_f_200msps_64i_4096c_adc_fmc1_g1/1 -> g1/1  "g1"
  g2_sim/1 -> snap2_f_200msps_64i_4096c_adc_fmc1_g2/1
  snap2_f_200msps_64i_4096c_adc_fmc1_g2/1 -> g2/1  "g2"
  g3_sim/1 -> snap2_f_200msps_64i_4096c_adc_fmc1_g3/1
  snap2_f_200msps_64i_4096c_adc_fmc1_g3/1 -> g3/1  "g3"
  g4_sim/1 -> snap2_f_200msps_64i_4096c_adc_fmc1_g4/1
  snap2_f_200msps_64i_4096c_adc_fmc1_g4/1 -> g4/1  "g4"
  h1_sim/1 -> snap2_f_200msps_64i_4096c_adc_fmc1_h1/1
  snap2_f_200msps_64i_4096c_adc_fmc1_h1/1 -> h1/1  "h1"
  h2_sim/1 -> snap2_f_200msps_64i_4096c_adc_fmc1_h2/1
  snap2_f_200msps_64i_4096c_adc_fmc1_h2/1 -> h2/1  "h2"
  h3_sim/1 -> snap2_f_200msps_64i_4096c_adc_fmc1_h3/1
  snap2_f_200msps_64i_4096c_adc_fmc1_h3/1 -> h3/1  "h3"
  h4_sim/1 -> snap2_f_200msps_64i_4096c_adc_fmc1_h4/1
  snap2_f_200msps_64i_4096c_adc_fmc1_h4/1 -> h4/1  "h4"
  sync/1 -> snap2_f_200msps_64i_4096c_adc_fmc1_adc_sync/1
  snap2_f_200msps_64i_4096c_adc_fmc1_adc_sync/1 -> sync_term/1
  rst/1 -> snap2_f_200msps_64i_4096c_adc_fmc1_adc_rst/1
  snap2_f_200msps_64i_4096c_adc_fmc1_adc_rst/1 -> rst_term/1
  snapshot_trig/1 -> snap2_f_200msps_64i_4096c_adc_fmc1_snapshot_ext_trigger/1
  snap2_f_200msps_64i_4096c_adc_fmc1_snapshot_ext_trigger/1 -> snapshot_trig_term/1
  sim_sync_out/1 -> snap2_f_200msps_64i_4096c_adc_fmc1_adc_sync_out/1
  snap2_f_200msps_64i_4096c_adc_fmc1_adc_sync_out/1 -> sync_out/1

== system snap2_f_200msps_64i_4096c/adc/sync ==
  sim_1 : Inport
  sim_2 : Inport  Port=2
  sim_3 : Inport  Port=3
  sim_4 : Inport  Port=4
  sim_5 : Inport  Port=5
  convert1_{1..5} (5 alike) : DataTypeConversion  OutDataTypeStr=fixdt('ufix1_En0')  LockScale=on
  convert2_{1..5} (5 alike) : DataTypeConversion  OutDataTypeStr=fixdt('ufix1_En0')  ConvertRealWorld=Stored Integer (SI)  LockScale=on
  gain_1 : Gain  Gain=16
  gain_2 : Gain  Gain=8
  gain_3 : Gain  Gain=4
  gain_4 : Gain  Gain=2
  gain_5 : Gain
  io_delay : xbsIndex_r4/Delay  rst=off  infoeditControl=Selection of Reset will increase slice count due to use of real FFs and instead of SRLs  en=off  latency=0  reg_retiming=on  dbl_ovrd=off  block_type=delay
  sim_add : Sum  Inputs=+++++  OutDataTypeStr=uint32
  slice_ext_ss_trig_en : xbsIndex_r4/Slice  nbits=1  boolean_output=on  mode=Lower Bit Location + Width  bit1=0  base1=MSB of Input  bit0=1  base0=LSB of Input  dbl_ovrd=off  block_type=slice
  slice_ext_sync_enable : xbsIndex_r4/Slice  nbits=1  boolean_output=on  mode=Lower Bit Location + Width  bit1=0  base1=MSB of Input  bit0=3  base0=LSB of Input  dbl_ovrd=off  block_type=slice
  slice_rst : xbsIndex_r4/Slice  nbits=1  boolean_output=on  mode=Lower Bit Location + Width  bit1=0  base1=MSB of Input  bit0=0  base0=LSB of Input  dbl_ovrd=off  block_type=slice
  slice_ss_trig : xbsIndex_r4/Slice  nbits=1  boolean_output=on  mode=Lower Bit Location + Width  bit1=0  base1=MSB of Input  bit0=2  base0=LSB of Input  dbl_ovrd=off  block_type=slice
  slice_sync : xbsIndex_r4/Slice  nbits=1  boolean_output=on  mode=Lower Bit Location + Width  bit1=0  base1=MSB of Input  bit0=4  base0=LSB of Input  dbl_ovrd=off  block_type=slice
  snap2_f_200msps_64i_4096c_adc_sync_user_data_out : xbsIndex_r4/Gateway In  gui_display_data_type=Fixed-point  arith_type=Unsigned  n_bits=32  bin_pt=0  preci_type=Single  exp_width=8  frac_width=24  rows=1  columns=1  quantization="Round  (unbiased: +/- Inf)"  overflow=Saturate  period=1  UseAsADC=off  ADCChannel='1'  interface=None  automatic_assignment=on  address_offset=hex2dec('00')  intf_name=''  intf_description=''  default_value=0  timing_constraint=None  locs_specified=off  LOCs={}  io_standard={}  inherit_from_input=off  hdl_port=on  dbl_ovrd=off  block_type=gatewayin
  in_sync : Outport
  in_ext_sync_enable : Outport  Port=2
  in_ss_trig : Outport  Port=3
  in_ext_ss_trig_en : Outport  Port=4
  in_rst : Outport  Port=5
  wires:
  snap2_f_200msps_64i_4096c_adc_sync_user_data_out/1 -> io_delay/1
  sim_add/1 -> snap2_f_200msps_64i_4096c_adc_sync_user_data_out/1
  sim_1/1 -> convert1_1/1
  convert1_1/1 -> convert2_1/1
  convert2_1/1 -> gain_1/1
  gain_1/1 -> sim_add/1
  io_delay/1 -> slice_sync/1, slice_ext_sync_enable/1, slice_ss_trig/1, slice_ext_ss_trig_en/1, slice_rst/1
  slice_sync/1 -> in_sync/1
  sim_2/1 -> convert1_2/1
  convert1_2/1 -> convert2_2/1
  convert2_2/1 -> gain_2/1
  gain_2/1 -> sim_add/2
  slice_ext_sync_enable/1 -> in_ext_sync_enable/1
  sim_3/1 -> convert1_3/1
  convert1_3/1 -> convert2_3/1
  convert2_3/1 -> gain_3/1
  gain_3/1 -> sim_add/3
  slice_ss_trig/1 -> in_ss_trig/1
  sim_4/1 -> convert1_4/1
  convert1_4/1 -> convert2_4/1
  convert2_4/1 -> gain_4/1
  gain_4/1 -> sim_add/4
  slice_ext_ss_trig_en/1 -> in_ext_ss_trig_en/1
  sim_5/1 -> convert1_5/1
  convert1_5/1 -> convert2_5/1
  convert2_5/1 -> gain_5/1
  gain_5/1 -> sim_add/5
  slice_rst/1 -> in_rst/1
